simulink model "psimulink"  (R2019a)
settings: Solver=VariableStepAuto  StartTime=0.0  StopTime=10.0  RelTol=1e-3
settings Model: Creator=acer  LastModifiedBy=acer

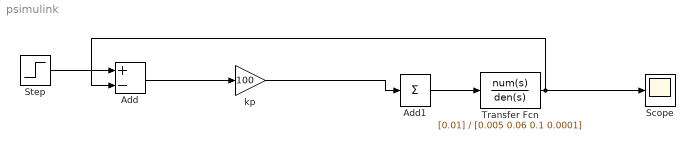
== system psimulink ==
  Add : Sum  Inputs=+-
  Add1 : Sum  Inputs=+
  Scope : Scope
  Step : Step  Time=0  SampleTime=0
  Transfer Fcn : TransferFcn  Numerator=[0.01]  Denominator=[0.005 0.06 0.1 0.0001]
  "kp " : Gain  Gain=100
  wires:
  Step/1 -> Add/1
  Add/1 -> "kp "/1
  "kp "/1 -> Add1/1
  Transfer Fcn/1 -> Add/2, Scope/1
  Add1/1 -> Transfer Fcn/1
